simulink model "QPSK_timing"  (R2016b)
settings: Solver=VariableStepAuto  StartTime=0.0  StopTime=(12+133)*8  RelTol=1e-3  EnableMultiTasking=on
undefined symbols (not defined in the file or in its folder): K1, K2, rcosine
libraries: simulink x5, dspstat3 x2, dspsigops x2, dspsrcs4 x1
settings Model: Creator=coltmt  LastModifiedBy=colttom
settings OptimizationCC: LifeSpan=inf
settings DebuggingCC: SFUnexpectedBacktrackingDiag=warning  SFNoUnconditionalDefaultTransitionDiag=warning  SFExecutionAtInitializationDiag=none
settings GRTTargetCC: TargetLangStandard=C89/C90 (ANSI)  GeneratePreprocessorConditionals=Disable all
settings ConfigComp: CovMetricSettings=dw  CovHtmlReporting=on  CovSaveCumulativeToWorkspaceVar=on  CovSaveSingleToWorkspaceVar=on  CovExternalEMLEnable=off

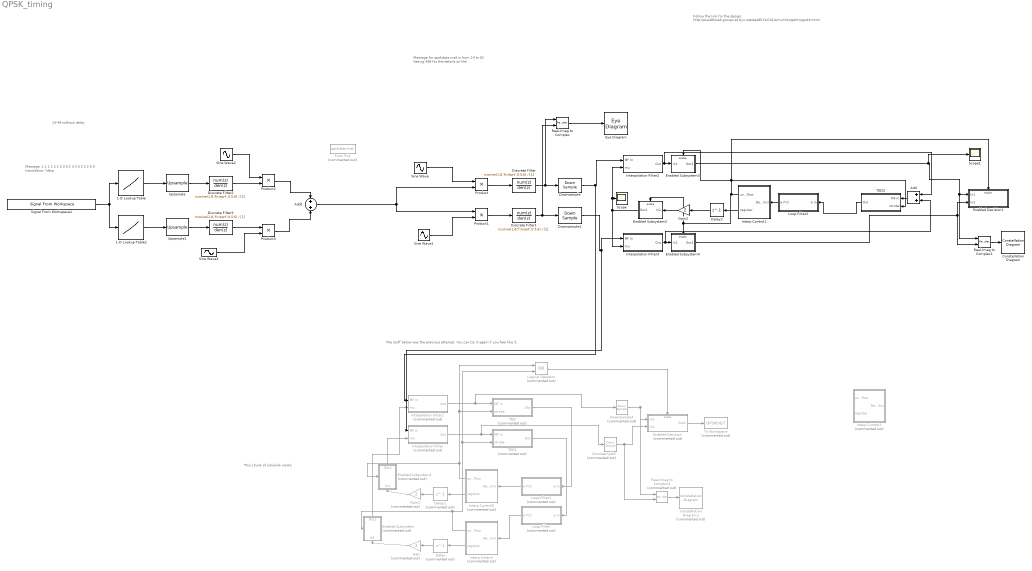
== system QPSK_timing ==
  note: This chunk of simulink works
  note: 13-48 without delay
  note: Message: 1 1 1 1 2 1 0 3 0 2 3 3 0 2 3 2 0 0
      | translation: *derp
  note: Follow the link for the design: http://ece485web.groups.et.byu.net/ee485.fall.01/simulink/qpsktr/qpsktr.html
  note: The stuff below was the previous attempt. You can try it again if you feel like it.
  note: Message for qpskdata.mat is from 14 to 62
      |
      | See pg 498 for the details on the
  1-D Lookup Table : Lookup_n-D  NumberOfTableDimensions=1  BreakpointsForDimension1=[0 1 2 3]  Table=[1 -1 1 -1]*3/sqrt(2)  InternalRulePriority=Speed  RndMeth=Simplest  InputSameDT=on
  1-D Lookup Table2 : Lookup_n-D  NumberOfTableDimensions=1  BreakpointsForDimension1=[0 1 2 3]  Table=[1 1 -1 -1]*3/sqrt(2)  InternalRulePriority=Speed  RndMeth=Simplest  InputSameDT=on
  Add : Sum
  Add1 : Sum
  Constellation Diagram : ConstellationDiagram
  Constellation Diagram1 : ConstellationDiagram  Commented=on
  Delay : Delay  Commented=on  DelayLength=1
  Delay1 : Delay  Commented=on  DelayLength=1
  Delay2 : Delay  DelayLength=1
  Discrete Filter{,1..3} (4 alike) : DiscreteFilter  Numerator=rcosine(1,8,'fir/sqrt',0.5,6)  Denominator=[1]
  Downsample : DownSample  N=16/2  phase=7  InputProcessing=Inherited (this choice will be removed - see release notes)  RateOptions=Allow multirate processing
  Downsample1 : DownSample  N=16/2  phase=7  InputProcessing=Inherited (this choice will be removed - see release notes)  RateOptions=Allow multirate processing
  Downsample4 : DownSample  Commented=on  RateOptions=Allow multirate processing
  Downsample5 : DownSample  Commented=on  RateOptions=Allow multirate processing
  Enabled Decision : Subsystem  Commented=on  TreatAsAtomicUnit=on
  Enabled Decision1 : Subsystem  TreatAsAtomicUnit=on
  Enabled Subsystem : Subsystem  Commented=on  TreatAsAtomicUnit=on
  Enabled Subsystem1 : Subsystem  Commented=on  TreatAsAtomicUnit=on
  Enabled Subsystem2 : Subsystem  TreatAsAtomicUnit=on
  Enabled Subsystem3 : Subsystem  TreatAsAtomicUnit=on
  Enabled Subsystem4 : Subsystem  TreatAsAtomicUnit=on
  Eye Diagram : EyeDiagram
  From File : FromFile  Commented=on  FileName=qpskdata.mat  SampleTime=1
  Gain : Gain  Commented=on  Gain=2
  Gain1 : Gain  Commented=on  Gain=2
  Gain2 : Gain  Gain=2
  Interp Control : Subsystem  Commented=on
  Interp Control1 : Subsystem
  Interp Control2 : Subsystem  Commented=on
  Interp Control3 : Subsystem  Commented=on
  Interpolation Filter : Subsystem  Commented=on
  Interpolation Filter1 : Subsystem  Commented=on
  Interpolation Filter2 : Subsystem
  Interpolation Filter3 : Subsystem
  Logical Operator : Logic  Commented=on  Operator=OR  AllPortsSameDT=off  OutDataTypeStr=boolean
  Loop Filter : Subsystem  Commented=on
  Loop Filter1 : Subsystem  Commented=on
  Loop Filter2 : Subsystem
  Product{,1..3} (4 alike) : Product
  Real-Imag to Complex : RealImagToComplex
  Real-Imag to Complex1 : RealImagToComplex
  Real-Imag to Complex2 : RealImagToComplex  Commented=on
  Scope : Scope
  Scope1 : Scope
  Signal From Workspace1 : dspsrcs4/Signal From Workspace  X=[1 2 3 0 0 2 3 1 3 2 1 0 3 2 0 2 0 1 4 2 3 1 0 2 3 1 2 3 0 3 2 1 2 3 0 2 3 3 1 2 3 1 2 3 1 2 3 1 2 1 2 1 2 2 1 2 1 2 1 2 1 2 1 2 1 2 1 2 1 2 1 0 0 3 2 0 1 2 0 1 3 2 3 1 1 1 1 1 0 0 0 1 1 0 0 1 1 1 1 2 1 0 3 0 2 3 3 0 2 3 2 0 0]  Ts=8  nsamps=1  OutputAfterFinalValue=Setting to zero  ignoreOrWarnInputAndFrameLengths=off  OutputFrames=off
  Sine Wave : Sin  Amplitude=sqrt(2)  Frequency=2*pi/4  Phase=pi/2  SampleTime=.5
  Sine Wave1 : Sin  Amplitude=-sqrt(2)  Frequency=2*pi/4  SampleTime=.5
  Sine Wave2 : Sin  Amplitude=sqrt(2)  Frequency=2*pi/4  Phase=pi/2  SampleTime=.5
  Sine Wave3 : Sin  Amplitude=-sqrt(2)  Frequency=2*pi/4  SampleTime=.5
  TED : Subsystem  Commented=on
  TED1 : Subsystem  Commented=on
  TED2 : Subsystem
  To Workspace : ToWorkspace  Commented=on  VariableName=QPSKbitsT  SampleTime=-1
      settings: Save2DSignal=2-D array (concatenate along first dimension)
  Upsample : dspsigops/Upsample  N=16  phase=0  InputProcessing=Inherited (this choice will be removed - see release notes)  RateOptions=Allow multirate processing  ic=0  mode=Unused parameter value
  Upsample1 : dspsigops/Upsample  N=16  phase=0  InputProcessing=Inherited (this choice will be removed - see release notes)  RateOptions=Allow multirate processing  ic=0  mode=Unused parameter value
  wires:
  Sine Wave1/1 -> Product1/2
  Sine Wave/1 -> Product/1
  Product1/1 -> Discrete Filter1/1
  Product/1 -> Discrete Filter/1
  Discrete Filter/1 -> Real-Imag to Complex/1, Downsample/1
  Discrete Filter1/1 -> Real-Imag to Complex/2, Downsample1/1
  Real-Imag to Complex/1 -> Eye Diagram/1
  Enabled Decision/1(Out1) -> To Workspace/1
  Interpolation Filter1/1(Out) -> Downsample4/1, TED/1(MF in)
  Interpolation Filter/1(Out) -> Downsample5/1, TED1/1(MF in)
  TED1/1(Out) -> Loop Filter/1(e in)
  TED/1(Out) -> Loop Filter1/1(e in)
  Loop Filter/1(e F(z)) -> Interp Control/1(Delta Incr)
  Loop Filter1/1(e F(z)) -> Interp Control3/1(Delta Incr)
  Interp Control/2(register) -> Delay/1
  Interp Control3/2(register) -> Delay1/1
  Delay/1 -> Gain/1
  Delay1/1 -> Gain1/1
  Gain/1 -> Enabled Subsystem/1(In1)
  Gain1/1 -> Enabled Subsystem1/1(In1)
  Enabled Subsystem1/1(Out1) -> Interpolation Filter/2(mu)
  Enabled Subsystem/1(Out1) -> Interpolation Filter1/2(mu)
  Interp Control/1(underflow) -> Enabled Subsystem/Enable, Logical Operator/2, TED1/2(strobe)
  Interp Control3/1(underflow) -> Logical Operator/1, TED/2(strobe), Enabled Subsystem1/Enable
  Logical Operator/1 -> Enabled Decision/Enable
  Downsample/1 -> Interpolation Filter1/1(MF In), Interpolation Filter2/1(MF In)
  Downsample1/1 -> Interpolation Filter/1(MF In), Interpolation Filter3/1(MF In)
  Loop Filter2/1(e F(z)) -> Interp Control1/1(Delta Incr)
  Interp Control1/2(register) -> Delay2/1
  Delay2/1 -> Gain2/1
  Gain2/1 -> Enabled Subsystem2/1(In1)
  Interp Control1/1(underflow) -> Enabled Decision1/Enable, TED2/2(strobe), Enabled Subsystem3/Enable, Enabled Subsystem4/Enable, Enabled Subsystem2/Enable
  Real-Imag to Complex1/1 -> Constellation Diagram/1
  Add/1 -> TED2/1(MF in)
  Interpolation Filter2/1(Out) -> Add/1, Enabled Subsystem3/1(In1)
  Interpolation Filter3/1(Out) -> Add/2, Enabled Subsystem4/1(In1)
  Enabled Subsystem2/1(Out1) -> Scope/1, Interpolation Filter2/2(mu), Interpolation Filter3/2(mu)
  Signal From Workspace1/1 -> 1-D Lookup Table2/1, 1-D Lookup Table/1
  1-D Lookup Table/1 -> Upsample/1
  1-D Lookup Table2/1 -> Upsample1/1
  Upsample/1 -> Discrete Filter2/1
  Upsample1/1 -> Discrete Filter3/1
  Discrete Filter2/1 -> Product2/2
  Sine Wave2/1 -> Product2/1
  Discrete Filter3/1 -> Product3/1
  Sine Wave3/1 -> Product3/2
  Product3/1 -> Add1/2
  Product2/1 -> Add1/1
  Enabled Subsystem3/1(Out1) -> Real-Imag to Complex1/1, Enabled Decision1/1(In1), Scope1/1
  Enabled Subsystem4/1(Out1) -> Enabled Decision1/2(In2), Real-Imag to Complex1/2
  Add1/1 -> Product/2, Product1/1
  Real-Imag to Complex2/1 -> Constellation Diagram1/1
  Downsample4/1 -> Real-Imag to Complex2/1, Enabled Decision/1(In1)
  Downsample5/1 -> Real-Imag to Complex2/2, Enabled Decision/2(In2)
  TED2/1(Out) -> Loop Filter2/1(e in)

== system QPSK_timing/Enabled Decision ==
  In1 : Inport
  In2 : Inport  Port=2
  Enable : EnablePort
  "QPSK decision " : Subsystem
  Out1 : Outport
  wires:
  "QPSK decision "/1(Out1) -> Out1/1
  In1/1 -> "QPSK decision "/1(In1)
  In2/1 -> "QPSK decision "/2(In2)

== system QPSK_timing/Enabled Decision1 ==
  In1 : Inport
  In2 : Inport  Port=2
  Enable : EnablePort
  "QPSK decision " : Subsystem
  To Workspace1 : ToWorkspace  VariableName=QPSKbitsT1  SampleTime=-1
      settings: Save2DSignal=2-D array (concatenate along first dimension)
  wires:
  "QPSK decision "/1(Out1) -> To Workspace1/1
  In1/1 -> "QPSK decision "/1(In1)
  In2/1 -> "QPSK decision "/2(In2)

== system QPSK_timing/Enabled Subsystem ==
  In1 : Inport
  Enable : EnablePort
  Out1 : Outport
  wires:
  In1/1 -> Out1/1

== system QPSK_timing/Enabled Subsystem1 ==
  In1 : Inport
  Enable : EnablePort
  Out1 : Outport
  wires:
  In1/1 -> Out1/1

== system QPSK_timing/Enabled Subsystem2 ==
  In1 : Inport
  Enable : EnablePort
  Out1 : Outport
  wires:
  In1/1 -> Out1/1

== system QPSK_timing/Enabled Subsystem3 ==
  In1 : Inport
  Enable : EnablePort
  Out1 : Outport
  wires:
  In1/1 -> Out1/1

== system QPSK_timing/Enabled Subsystem4 ==
  In1 : Inport
  Enable : EnablePort
  Out1 : Outport
  wires:
  In1/1 -> Out1/1

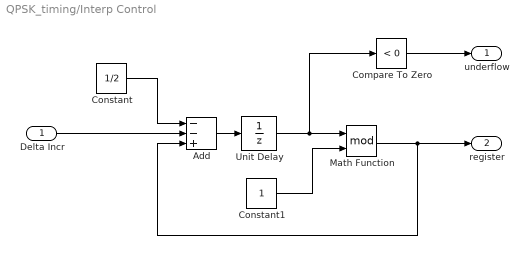
== system QPSK_timing/Interp Control ==
  Delta Incr : Inport
  Add : Sum  Inputs=--+
  Compare To Zero : simulink/Logic and Bit Operations/Compare To Zero  relop=<  OutDataTypeStr=boolean
  Constant : Constant  Value=1/2
  Constant1 : Constant
  Math Function : Math  Operator=mod  SaturateOnIntegerOverflow=on
  Unit Delay : UnitDelay  SampleTime=-1
  underflow : Outport
  register : Outport  Port=2
  wires:
  Delta Incr/1 -> Add/2
  Constant/1 -> Add/1
  Add/1 -> Unit Delay/1
  Constant1/1 -> Math Function/2
  Unit Delay/1 -> Compare To Zero/1, Math Function/1
  Math Function/1 -> Add/3, register/1
  Compare To Zero/1 -> underflow/1

== system QPSK_timing/Interp Control1 ==
  Delta Incr : Inport
  Add : Sum  Inputs=--+
  Compare To Zero : simulink/Logic and Bit Operations/Compare To Zero  relop=<  OutDataTypeStr=boolean
  Constant : Constant  Value=1/2
  Constant1 : Constant
  Math Function : Math  Operator=mod  SaturateOnIntegerOverflow=on
  Unit Delay : UnitDelay  SampleTime=-1
  underflow : Outport
  register : Outport  Port=2
  wires:
  Delta Incr/1 -> Add/2
  Constant/1 -> Add/1
  Add/1 -> Unit Delay/1
  Constant1/1 -> Math Function/2
  Unit Delay/1 -> Compare To Zero/1, Math Function/1
  Math Function/1 -> Add/3, register/1
  Compare To Zero/1 -> underflow/1

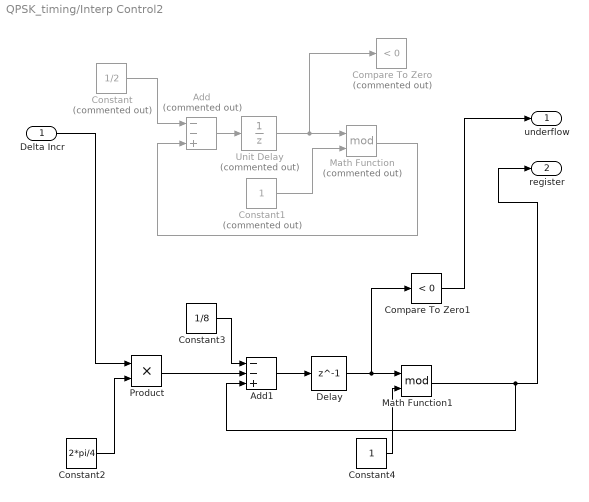
== system QPSK_timing/Interp Control2 ==
  Delta Incr : Inport
  Add : Sum  Commented=on  Inputs=--+
  Add1 : Sum  Inputs=--+
  Compare To Zero : simulink/Logic and Bit Operations/Compare To Zero  Commented=on  relop=<  OutDataTypeStr=boolean
  Compare To Zero1 : simulink/Logic and Bit Operations/Compare To Zero  relop=<  OutDataTypeStr=boolean
  Constant : Constant  Commented=on  Value=1/2
  Constant1 : Constant  Commented=on
  Constant2 : Constant  Value=2*pi/4
  Constant3 : Constant  Value=1/8
  Constant4 : Constant
  Delay : Delay  DelayLength=1
  Math Function : Math  Commented=on  Operator=mod  SaturateOnIntegerOverflow=on
  Math Function1 : Math  Operator=mod  SaturateOnIntegerOverflow=on
  Product : Product
  Unit Delay : UnitDelay  Commented=on  SampleTime=-1
  underflow : Outport
  register : Outport  Port=2
  wires:
  Constant/1 -> Add/1
  Add/1 -> Unit Delay/1
  Constant1/1 -> Math Function/2
  Unit Delay/1 -> Compare To Zero/1, Math Function/1
  Math Function/1 -> Add/3
  Constant2/1 -> Product/2
  Product/1 -> Add1/2
  Constant3/1 -> Add1/1
  Add1/1 -> Delay/1
  Delay/1 -> Compare To Zero1/1, Math Function1/1
  Constant4/1 -> Math Function1/2
  Math Function1/1 -> Add1/3, register/1
  Delta Incr/1 -> Product/1
  Compare To Zero1/1 -> underflow/1

== system QPSK_timing/Interp Control3 ==
  Delta Incr : Inport
  Add : Sum  Inputs=--+
  Compare To Zero : simulink/Logic and Bit Operations/Compare To Zero  relop=<  OutDataTypeStr=boolean
  Constant : Constant  Value=1/2
  Constant1 : Constant
  Math Function : Math  Operator=mod  SaturateOnIntegerOverflow=on
  Unit Delay : UnitDelay  SampleTime=-1
  underflow : Outport
  register : Outport  Port=2
  wires:
  Delta Incr/1 -> Add/2
  Constant/1 -> Add/1
  Add/1 -> Unit Delay/1
  Constant1/1 -> Math Function/2
  Unit Delay/1 -> Compare To Zero/1, Math Function/1
  Math Function/1 -> Add/3, register/1
  Compare To Zero/1 -> underflow/1

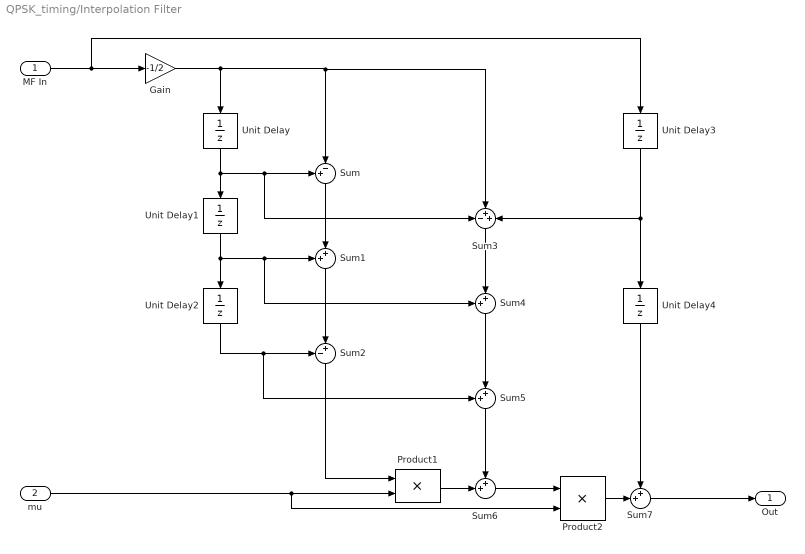
== system QPSK_timing/Interpolation Filter ==
  MF In : Inport
  mu : Inport  Port=2
  Gain : Gain  Gain=-1/2
  Product1 : Product  SaturateOnIntegerOverflow=on  InputSameDT=on  OutDataTypeStr=Inherit: Same as first input
  Product2 : Product  SaturateOnIntegerOverflow=on  InputSameDT=on  OutDataTypeStr=Inherit: Same as first input
  Sum : Sum  Inputs=+-|  SaturateOnIntegerOverflow=on  InputSameDT=on  OutDataTypeStr=Inherit: Same as first input
  Sum{1,4..7} (5 alike) : Sum  Inputs=++|  SaturateOnIntegerOverflow=on  InputSameDT=on  OutDataTypeStr=Inherit: Same as first input
  Sum2 : Sum  Inputs=-+|  SaturateOnIntegerOverflow=on  InputSameDT=on  OutDataTypeStr=Inherit: Same as first input
  Sum3 : Sum  Inputs=-++  SaturateOnIntegerOverflow=on  InputSameDT=on  OutDataTypeStr=Inherit: Same as first input
  Unit Delay{,1..4} (5 alike) : UnitDelay  SampleTime=-1
  Out : Outport
  wires:
  Sum1/1 -> Sum2/2
  Sum/1 -> Sum1/2
  Unit Delay/1 -> Sum3/1, Sum/1, Unit Delay1/1
  Unit Delay1/1 -> Sum4/1, Sum1/1, Unit Delay2/1
  Unit Delay2/1 -> Sum5/1, Sum2/1
  Sum5/1 -> Sum6/1
  Product1/1 -> Sum6/2
  Sum4/1 -> Sum5/2
  Sum3/1 -> Sum4/2
  MF In/1 -> Unit Delay3/1, Gain/1
  Gain/1 -> Unit Delay/1, Sum/2, Sum3/2
  Product2/1 -> Sum7/2
  Unit Delay4/1 -> Sum7/1
  Sum6/1 -> Product2/1
  Sum7/1 -> Out/1
  Unit Delay3/1 -> Sum3/3, Unit Delay4/1
  Sum2/1 -> Product1/1
  mu/1 -> Product2/2, Product1/2

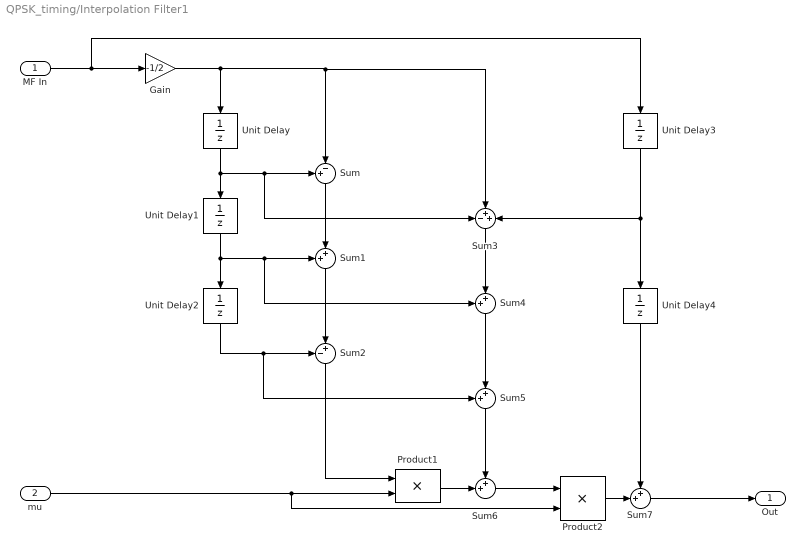
== system QPSK_timing/Interpolation Filter1 ==
  MF In : Inport
  mu : Inport  Port=2
  Gain : Gain  Gain=-1/2
  Product1 : Product  SaturateOnIntegerOverflow=on  InputSameDT=on  OutDataTypeStr=Inherit: Same as first input
  Product2 : Product  SaturateOnIntegerOverflow=on  InputSameDT=on  OutDataTypeStr=Inherit: Same as first input
  Sum : Sum  Inputs=+-|  SaturateOnIntegerOverflow=on  InputSameDT=on  OutDataTypeStr=Inherit: Same as first input
  Sum{1,4..7} (5 alike) : Sum  Inputs=++|  SaturateOnIntegerOverflow=on  InputSameDT=on  OutDataTypeStr=Inherit: Same as first input
  Sum2 : Sum  Inputs=-+|  SaturateOnIntegerOverflow=on  InputSameDT=on  OutDataTypeStr=Inherit: Same as first input
  Sum3 : Sum  Inputs=-++  SaturateOnIntegerOverflow=on  InputSameDT=on  OutDataTypeStr=Inherit: Same as first input
  Unit Delay{,1..4} (5 alike) : UnitDelay  SampleTime=-1
  Out : Outport
  wires:
  Sum1/1 -> Sum2/2
  Sum/1 -> Sum1/2
  Unit Delay/1 -> Sum3/1, Sum/1, Unit Delay1/1
  Unit Delay1/1 -> Sum4/1, Sum1/1, Unit Delay2/1
  Unit Delay2/1 -> Sum5/1, Sum2/1
  Sum5/1 -> Sum6/1
  Product1/1 -> Sum6/2
  Sum4/1 -> Sum5/2
  Sum3/1 -> Sum4/2
  MF In/1 -> Unit Delay3/1, Gain/1
  Gain/1 -> Unit Delay/1, Sum/2, Sum3/2
  Product2/1 -> Sum7/2
  Unit Delay4/1 -> Sum7/1
  Sum6/1 -> Product2/1
  Sum7/1 -> Out/1
  Unit Delay3/1 -> Sum3/3, Unit Delay4/1
  Sum2/1 -> Product1/1
  mu/1 -> Product2/2, Product1/2

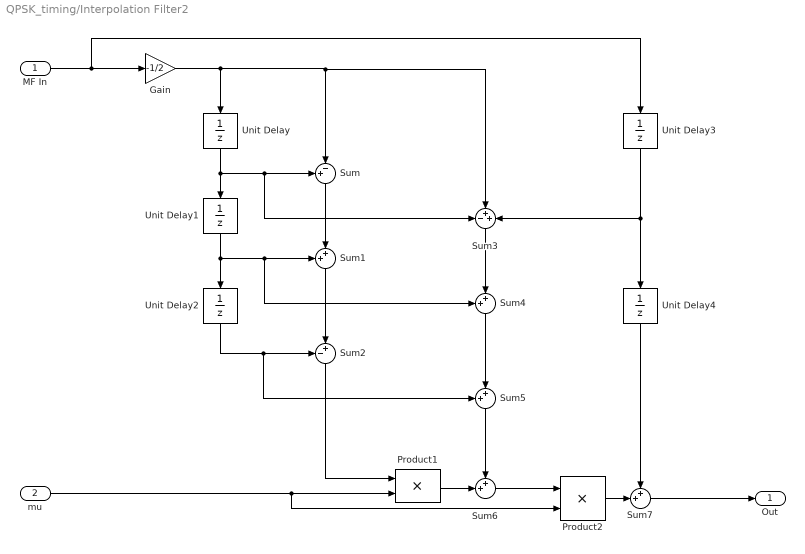
== system QPSK_timing/Interpolation Filter2 ==
  MF In : Inport
  mu : Inport  Port=2
  Gain : Gain  Gain=-1/2
  Product1 : Product  SaturateOnIntegerOverflow=on  InputSameDT=on  OutDataTypeStr=Inherit: Same as first input
  Product2 : Product  SaturateOnIntegerOverflow=on  InputSameDT=on  OutDataTypeStr=Inherit: Same as first input
  Sum : Sum  Inputs=+-|  SaturateOnIntegerOverflow=on  InputSameDT=on  OutDataTypeStr=Inherit: Same as first input
  Sum{1,4..7} (5 alike) : Sum  Inputs=++|  SaturateOnIntegerOverflow=on  InputSameDT=on  OutDataTypeStr=Inherit: Same as first input
  Sum2 : Sum  Inputs=-+|  SaturateOnIntegerOverflow=on  InputSameDT=on  OutDataTypeStr=Inherit: Same as first input
  Sum3 : Sum  Inputs=-++  SaturateOnIntegerOverflow=on  InputSameDT=on  OutDataTypeStr=Inherit: Same as first input
  Unit Delay{,1..4} (5 alike) : UnitDelay  SampleTime=-1
  Out : Outport
  wires:
  Sum1/1 -> Sum2/2
  Sum/1 -> Sum1/2
  Unit Delay/1 -> Sum3/1, Sum/1, Unit Delay1/1
  Unit Delay1/1 -> Sum4/1, Sum1/1, Unit Delay2/1
  Unit Delay2/1 -> Sum5/1, Sum2/1
  Sum5/1 -> Sum6/1
  Product1/1 -> Sum6/2
  Sum4/1 -> Sum5/2
  Sum3/1 -> Sum4/2
  MF In/1 -> Unit Delay3/1, Gain/1
  Gain/1 -> Unit Delay/1, Sum/2, Sum3/2
  Product2/1 -> Sum7/2
  Unit Delay4/1 -> Sum7/1
  Sum6/1 -> Product2/1
  Sum7/1 -> Out/1
  Unit Delay3/1 -> Sum3/3, Unit Delay4/1
  Sum2/1 -> Product1/1
  mu/1 -> Product2/2, Product1/2

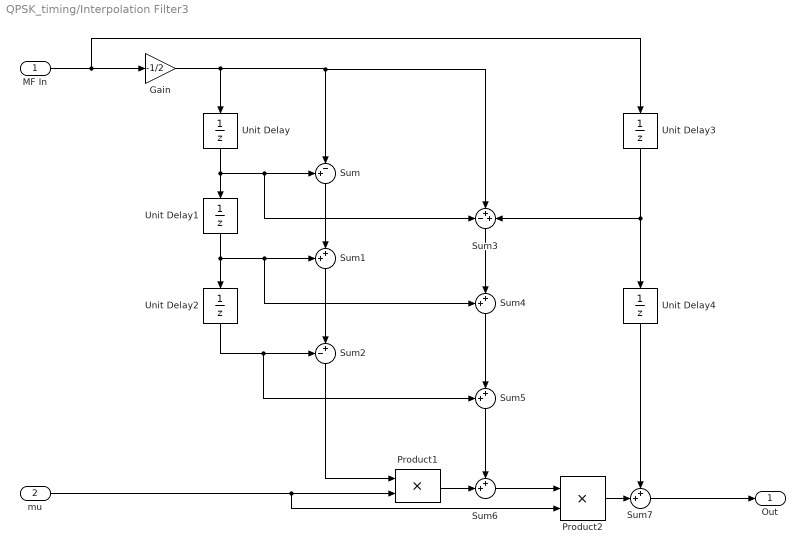
== system QPSK_timing/Interpolation Filter3 ==
  MF In : Inport
  mu : Inport  Port=2
  Gain : Gain  Gain=-1/2
  Product1 : Product  SaturateOnIntegerOverflow=on  InputSameDT=on  OutDataTypeStr=Inherit: Same as first input
  Product2 : Product  SaturateOnIntegerOverflow=on  InputSameDT=on  OutDataTypeStr=Inherit: Same as first input
  Sum : Sum  Inputs=+-|  SaturateOnIntegerOverflow=on  InputSameDT=on  OutDataTypeStr=Inherit: Same as first input
  Sum{1,4..7} (5 alike) : Sum  Inputs=++|  SaturateOnIntegerOverflow=on  InputSameDT=on  OutDataTypeStr=Inherit: Same as first input
  Sum2 : Sum  Inputs=-+|  SaturateOnIntegerOverflow=on  InputSameDT=on  OutDataTypeStr=Inherit: Same as first input
  Sum3 : Sum  Inputs=-++  SaturateOnIntegerOverflow=on  InputSameDT=on  OutDataTypeStr=Inherit: Same as first input
  Unit Delay{,1..4} (5 alike) : UnitDelay  SampleTime=-1
  Out : Outport
  wires:
  Sum1/1 -> Sum2/2
  Sum/1 -> Sum1/2
  Unit Delay/1 -> Sum3/1, Sum/1, Unit Delay1/1
  Unit Delay1/1 -> Sum4/1, Sum1/1, Unit Delay2/1
  Unit Delay2/1 -> Sum5/1, Sum2/1
  Sum5/1 -> Sum6/1
  Product1/1 -> Sum6/2
  Sum4/1 -> Sum5/2
  Sum3/1 -> Sum4/2
  MF In/1 -> Unit Delay3/1, Gain/1
  Gain/1 -> Unit Delay/1, Sum/2, Sum3/2
  Product2/1 -> Sum7/2
  Unit Delay4/1 -> Sum7/1
  Sum6/1 -> Product2/1
  Sum7/1 -> Out/1
  Unit Delay3/1 -> Sum3/3, Unit Delay4/1
  Sum2/1 -> Product1/1
  mu/1 -> Product2/2, Product1/2

== system QPSK_timing/Loop Filter ==
  e in : Inport
  Discrete Filter : DiscreteFilter  Numerator=[(K1+K2) -K1]  Denominator=[1 -1]
  e F(z) : Outport
  wires:
  e in/1 -> Discrete Filter/1
  Discrete Filter/1 -> e F(z)/1

== system QPSK_timing/Loop Filter1 ==
  e in : Inport
  Discrete Filter : DiscreteFilter  Numerator=[(K1+K2) -K1]  Denominator=[1 -1]
  e F(z) : Outport
  wires:
  e in/1 -> Discrete Filter/1
  Discrete Filter/1 -> e F(z)/1

== system QPSK_timing/Loop Filter2 ==
  e in : Inport
  Discrete Filter : DiscreteFilter  Numerator=[(K1+K2) -K1]  Denominator=[1 -1]
  e F(z) : Outport
  wires:
  e in/1 -> Discrete Filter/1
  Discrete Filter/1 -> e F(z)/1

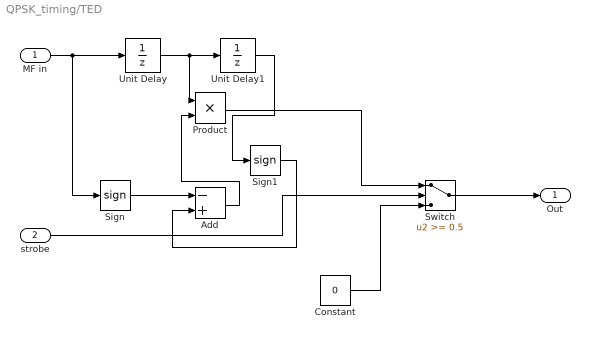
== system QPSK_timing/TED ==
  MF in : Inport
  strobe : Inport  Port=2
  Add : Sum  Inputs=-+
  Constant : Constant  Value=0
  Product : Product
  Sign : Signum
  Sign1 : Signum
  Switch : Switch  Threshold=0.5  SaturateOnIntegerOverflow=on
  Unit Delay : UnitDelay  SampleTime=-1
  Unit Delay1 : UnitDelay  SampleTime=-1
  Out : Outport
  wires:
  Switch/1 -> Out/1
  Constant/1 -> Switch/3
  strobe/1 -> Switch/2
  MF in/1 -> Sign/1, Unit Delay/1
  Unit Delay/1 -> Product/1, Unit Delay1/1
  Sign/1 -> Add/1
  Add/1 -> Product/2
  Unit Delay1/1 -> Sign1/1
  Sign1/1 -> Add/2
  Product/1 -> Switch/1

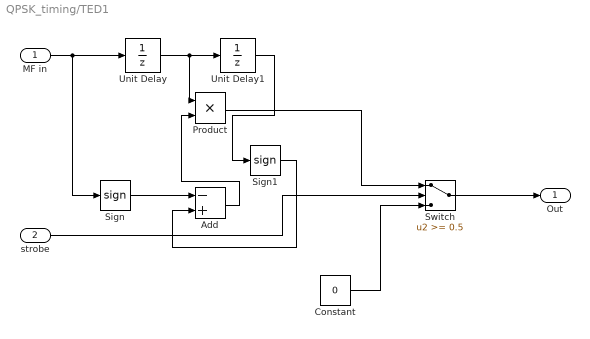
== system QPSK_timing/TED1 ==
  MF in : Inport
  strobe : Inport  Port=2
  Add : Sum  Inputs=-+
  Constant : Constant  Value=0
  Product : Product
  Sign : Signum
  Sign1 : Signum
  Switch : Switch  Threshold=0.5  SaturateOnIntegerOverflow=on
  Unit Delay : UnitDelay  SampleTime=-1
  Unit Delay1 : UnitDelay  SampleTime=-1
  Out : Outport
  wires:
  Switch/1 -> Out/1
  Constant/1 -> Switch/3
  strobe/1 -> Switch/2
  MF in/1 -> Sign/1, Unit Delay/1
  Unit Delay/1 -> Product/1, Unit Delay1/1
  Sign/1 -> Add/1
  Add/1 -> Product/2
  Unit Delay1/1 -> Sign1/1
  Sign1/1 -> Add/2
  Product/1 -> Switch/1

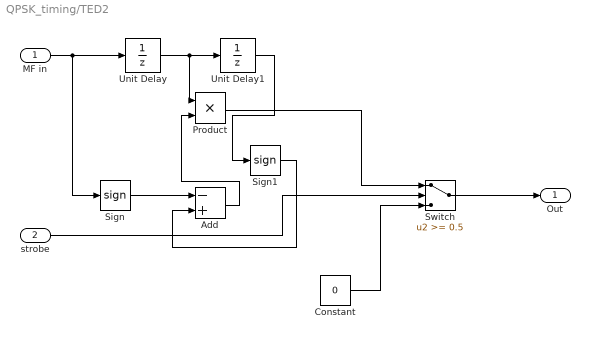
== system QPSK_timing/TED2 ==
  MF in : Inport
  strobe : Inport  Port=2
  Add : Sum  Inputs=-+
  Constant : Constant  Value=0
  Product : Product
  Sign : Signum
  Sign1 : Signum
  Switch : Switch  Threshold=0.5  SaturateOnIntegerOverflow=on
  Unit Delay : UnitDelay  SampleTime=-1
  Unit Delay1 : UnitDelay  SampleTime=-1
  Out : Outport
  wires:
  Switch/1 -> Out/1
  Constant/1 -> Switch/3
  strobe/1 -> Switch/2
  MF in/1 -> Sign/1, Unit Delay/1
  Unit Delay/1 -> Product/1, Unit Delay1/1
  Sign/1 -> Add/1
  Add/1 -> Product/2
  Unit Delay1/1 -> Sign1/1
  Sign1/1 -> Add/2
  Product/1 -> Switch/1

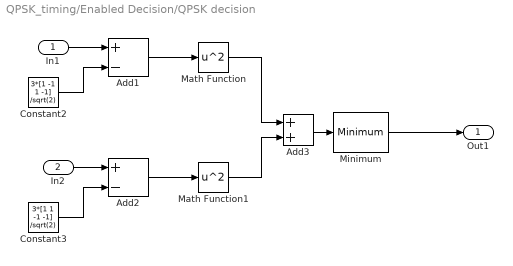
== system QPSK_timing/Enabled Decision/QPSK decision  ==
  In1 : Inport
  In2 : Inport  Port=2
  Add1 : Sum  Inputs=+-
  Add2 : Sum  Inputs=+-
  Add3 : Sum
  Constant2 : Constant  Value=3*[1 -1 1 -1] /sqrt(2)
  Constant3 : Constant  Value=3*[1 1 -1 -1] /sqrt(2)
  Math Function : Math  Operator=square  SaturateOnIntegerOverflow=on
  Math Function1 : Math  Operator=square  SaturateOnIntegerOverflow=on
  Minimum : dspstat3/Minimum  fcn=Index  reset=None  InputProcessing=Columns as channels (frame based)  indexBase=Zero  operateOver=Each column  Dimension=1  operation=minimum  roiEnable=off  roiType=Rectangles  roiPortion=Entire ROI  roiOutput=Individual statistics for each ROI  roiFlag=off  roundingMode=Floor  overflowMode=off
  Out1 : Outport
  wires:
  Math Function/1 -> Add3/1
  Math Function1/1 -> Add3/2
  Add3/1 -> Minimum/1
  Minimum/1 -> Out1/1
  Add1/1 -> Math Function/1
  Add2/1 -> Math Function1/1
  Constant3/1 -> Add2/2
  Constant2/1 -> Add1/2
  In1/1 -> Add1/1
  In2/1 -> Add2/1

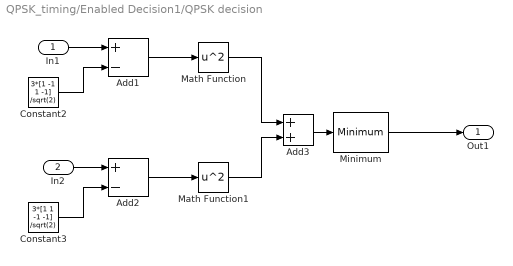
== system QPSK_timing/Enabled Decision1/QPSK decision  ==
  In1 : Inport
  In2 : Inport  Port=2
  Add1 : Sum  Inputs=+-
  Add2 : Sum  Inputs=+-
  Add3 : Sum
  Constant2 : Constant  Value=3*[1 -1 1 -1] /sqrt(2)
  Constant3 : Constant  Value=3*[1 1 -1 -1] /sqrt(2)
  Math Function : Math  Operator=square  SaturateOnIntegerOverflow=on
  Math Function1 : Math  Operator=square  SaturateOnIntegerOverflow=on
  Minimum : dspstat3/Minimum  operation=minimum  fcn=Index  indexBase=Zero  operateOver=Each column  Dimension=1  InputProcessing=Columns as channels (frame based)  reset=None  roiEnable=off  roiType=Rectangles  roiPortion=Entire ROI  roiOutput=Individual statistics for each ROI  roiFlag=off  roundingMode=Floor  overflowMode=off
  Out1 : Outport
  wires:
  Math Function/1 -> Add3/1
  Math Function1/1 -> Add3/2
  Add3/1 -> Minimum/1
  Minimum/1 -> Out1/1
  Add1/1 -> Math Function/1
  Add2/1 -> Math Function1/1
  Constant3/1 -> Add2/2
  Constant2/1 -> Add1/2
  In1/1 -> Add1/1
  In2/1 -> Add2/1
